simulink model "IKTrajectoryControlExamplechangepoints_MechanicalArm"  (R2019b)
settings: Solver=ode3  StartTime=0.0  StopTime=10  FixedStep=Ts  RelTol=1e-3
PostLoadFcn:
  | robot=importrobot('demo.urdf');
  | robot.DataFormat = 'column';
  | 
  | I = imread('coins.png');
  | imageOrigin = [40,20,0.08];
  | scale = .15;
model workspace (MAT data in the model file):
  I = [49 47 48 48 48 48 48 51 50 51 50 47 ... (73800 elements, 246x300)]
  Ts = 0.01
  filterConst = 0.08
  force_range = [0.8 0.9]
  imageOrigin = [0.4 0.2 0.08]
  initTargetPose = [-1  0  1.22464679915e-16  0.4; 0  1  0  0.2; -1.22464679915e-16  0  -1  0.28; 0  0  0  1]
  q0 = [0.422405030154; 0; -1.22880122285; 0]
  robot = robotics.RigidBodyTree
  robot.TreeInternal = robotics.manip.internal.RigidBodyTree
  robot.TreeInternal.NumBodies = 4
  robot.TreeInternal.Base = robotics.manip.internal.RigidBody
  robot.TreeInternal.Base.Index = 0
  robot.TreeInternal.Base.NameInternal = 'base_link'
  robot.TreeInternal.Base.JointInternal = robotics.Joint
  robot.TreeInternal.Base.JointInternal.Type = 'fixed'
  robot.TreeInternal.Base.JointInternal.VelocityNumber = 0
  robot.TreeInternal.Base.JointInternal.PositionNumber = 0
  robot.TreeInternal.Base.JointInternal.MotionSubspace = [0; 0; 0; 0; 0; 0]
  robot.TreeInternal.Base.JointInternal.NameInternal = 'base_link_jnt'
  robot.TreeInternal.Base.ParentIndex = -1
  robot.TreeInternal.Base.ChildrenIndices = 1
  robot.TreeInternal.Base.MassInternal = 60.86397744
  robot.TreeInternal.Base.CenterOfMassInternal = [0 0 0]
  robot.TreeInternal.Base.InertiaInternal = [5.0635929  0.00103417  0.80199628; 0.00103417  6.08689388  0.00105311; 0.80199628  0.00105311  4.96191932]
  robot.TreeInternal.Base.SpatialInertia = [5.0635929  0.00103417  0.80199628  0  0  0; 0.00103417  6.08689388  0.00105311  0  0  0; 0.80199628  0.00105311  4.96191932  0  0  0; 0  0  0  60.86397744  0  0; 0  0  0  0  60.86397744  0; 0  0  0  0  0  60.86397744]
  robot.TreeInternal.Base.VisualsInternal{1} = robotics.manip.internal.RigidBodyGeometry
  robot.TreeInternal.Base.VisualsInternal{1}.SourceData = {'Mesh', 'C:\Users\xxoo\Desktop\齐鹏老师\程序源码\TrajectoryControlThroughInverseKinematicsExample\magician\meshes\base_link.STL'}
  robot.TreeInternal.Base.VisualsInternal{1}.Vertices = [0.0640000030398 0.0640000030398 -0.0640000030398 -0.0640000030398 -0.0686352550983 -0.0686352550983 -0.0688218101859 -0.0640000030398 0.0686352550983 0.0640000030398 -0.0640000030398 0.0640000030398 ... (13851 elements, 4617x3)]
  robot.TreeInternal.Base.VisualsInternal{1}.Faces = [1 2 5 4 6 7 8 9 8 10 11 12 ... (28218 elements, 9406x3)]
  robot.TreeInternal.Base.VisualsInternal{1}.Color = [1 1 1 1]
  robot.TreeInternal.Base.VisualsInternal{1}.Tform = [1  0  0  0; 0  1  0  0; 0  0  1  0; 0  0  0  1]
  robot.TreeInternal.Gravity = [0 0 0]
  robot.TreeInternal.Bodies{1} = robotics.manip.internal.RigidBody
  robot.TreeInternal.Bodies{1}.Index = 1
  robot.TreeInternal.Bodies{1}.NameInternal = 'link_1'
  robot.TreeInternal.Bodies{1}.JointInternal = robotics.Joint
  robot.TreeInternal.Bodies{1}.JointInternal.Type = 'revolute'
  robot.TreeInternal.Bodies{1}.JointInternal.VelocityNumber = 1
  robot.TreeInternal.Bodies{1}.JointInternal.PositionNumber = 1
  robot.TreeInternal.Bodies{1}.JointInternal.MotionSubspace = [0; 0; 1; 0; 0; 0]
  robot.TreeInternal.Bodies{1}.JointInternal.InTree = 1
  robot.TreeInternal.Bodies{1}.JointInternal.JointToParentTransform = [1  0  0  0; 0  1  0  0; 0  0  1  0.024; 0  0  0  1]
  robot.TreeInternal.Bodies{1}.JointInternal.NameInternal = 'joint_1'
  robot.TreeInternal.Bodies{1}.JointInternal.PositionLimitsInternal = [-3.14159265 3.14159265]
  robot.TreeInternal.Bodies{1}.JointInternal.JointAxisInternal = [0 0 1]
  robot.TreeInternal.Bodies{1}.ParentIndex = 0
  robot.TreeInternal.Bodies{1}.ChildrenIndices = [0 1]
  robot.TreeInternal.Bodies{1}.MassInternal = 2.0687
  robot.TreeInternal.Bodies{1}.CenterOfMassInternal = [-0.0006241 -2.8025e-05 0.065404]
  robot.TreeInternal.Bodies{1}.InertiaInternal = [0.0156091448937  -4.20601823957e-05  8.38224731207e-05; -4.20601823957e-05  0.0156377490293  1.96798176658e-05; 8.38224731207e-05  1.96798176658e-05  0.00740390738508]
  robot.TreeInternal.Bodies{1}.SpatialInertia = [0.0156091448937  -4.20601823957e-05  8.38224731207e-05  0  -0.1353012548  -5.79753175e-05; -4.20601823957e-05  0.0156377490293  1.96798176658e-05  0.1353012548  0  0.00129107567; 8.38224731207e-05  1.96798176658e-05  0.00740390738508  5.79753175e-05  -0.00129107567  0; 0  0.1353012548  5.79753175e-05  2.0687  0  0; -0.1353012548  0  -0.00129107567  0  2.0687  0; -5.79753175e-05  0.00129107567  0  0  0  2.0687]
  robot.TreeInternal.Bodies{1}.VisualsInternal{1} = robotics.manip.internal.RigidBodyGeometry
  robot.TreeInternal.Bodies{1}.VisualsInternal{1}.SourceData = {'Mesh', 'C:\Users\xxoo\Desktop\齐鹏老师\程序源码\TrajectoryControlThroughInverseKinematicsExample\magician\meshes\link_1.STL'}
  robot.TreeInternal.Bodies{1}.VisualsInternal{1}.Vertices = [-0.0161934196949 -0.0211831368506 -0.0211831368506 -0.0161934196949 -0.0211167745292 -0.0211167745292 -0.0161065105349 0.0211831368506 -0.0083934366703 -0.0083934366703 -0.0161065105349 0.0161934196949 ... (4779 elements, 1593x3)]
  robot.TreeInternal.Bodies{1}.VisualsInternal{1}.Faces = [1 4 5 2 6 7 8 5 9 10 8 5 ... (9570 elements, 3190x3)]
  robot.TreeInternal.Bodies{1}.VisualsInternal{1}.Tform = [1  0  0  0; 0  1  0  0; 0  0  1  0; 0  0  0  1]
  robot.TreeInternal.Bodies{2} = robotics.manip.internal.RigidBody
  robot.TreeInternal.Bodies{2}.Index = 2
  robot.TreeInternal.Bodies{2}.NameInternal = 'link_2'
  robot.TreeInternal.Bodies{2}.JointInternal = robotics.Joint
  robot.TreeInternal.Bodies{2}.JointInternal.Type = 'revolute'
  robot.TreeInternal.Bodies{2}.JointInternal.VelocityNumber = 1
  robot.TreeInternal.Bodies{2}.JointInternal.PositionNumber = 1
  robot.TreeInternal.Bodies{2}.JointInternal.MotionSubspace = [0; 0; 1; 0; 0; 0]
  robot.TreeInternal.Bodies{2}.JointInternal.InTree = 1
  robot.TreeInternal.Bodies{2}.JointInternal.JointToParentTransform = [1.79489651492e-09  1.79489651492e-09  -1  -0.01175; -1  3.22165349927e-18  -1.79489651492e-09  0; 0  1  1.79489651492e-09  0.114; 0  0  0  1]
  robot.TreeInternal.Bodies{2}.JointInternal.NameInternal = 'joint_2'
  robot.TreeInternal.Bodies{2}.JointInternal.PositionLimitsInternal = [0 1.570796325]
  robot.TreeInternal.Bodies{2}.JointInternal.JointAxisInternal = [0 0 1]
  robot.TreeInternal.Bodies{2}.ParentIndex = 1
  robot.TreeInternal.Bodies{2}.ChildrenIndices = [0 0 1]
  robot.TreeInternal.Bodies{2}.MassInternal = 5.3213
  robot.TreeInternal.Bodies{2}.CenterOfMassInternal = [0.024366 0.010969 0.14363]
  robot.TreeInternal.Bodies{2}.InertiaInternal = [0.163730420845  0.00328707266887  -0.00688889284075; 0.00328707266887  0.170837433776  -0.000365688261111; -0.00688889284075  -0.000365688261111  0.0274585195056]
  robot.TreeInternal.Bodies{2}.SpatialInertia = [0.163730420845  0.00328707266887  -0.00688889284075  0  -0.764298319  0.0583693397; 0.00328707266887  0.170837433776  -0.000365688261111  0.764298319  0  -0.1296587958; -0.00688889284075  -0.000365688261111  0.0274585195056  -0.0583693397  0.1296587958  0; 0  0.764298319  -0.0583693397  5.3213  0  0; -0.764298319  0  0.1296587958  0  5.3213  0; 0.0583693397  -0.1296587958  0  0  0  5.3213]
  robot.TreeInternal.Bodies{2}.VisualsInternal{1} = robotics.manip.internal.RigidBodyGeometry
  robot.TreeInternal.Bodies{2}.VisualsInternal{1}.SourceData = {'Mesh', 'C:\Users\xxoo\Desktop\齐鹏老师\程序源码\TrajectoryControlThroughInverseKinematicsExample\magician\meshes\link_2.STL'}
  robot.TreeInternal.Bodies{2}.VisualsInternal{1}.Vertices = [0.0111309718341 0.0105486791581 0.0104152234271 0.0111560225487 0.0105787822977 0.0104152234271 0.0105787822977 0.0109527166933 0.0105486791581 0.0111309718341 0.0113159539178 0.0109527166933 ... (12384 elements, 4128x3)]
  robot.TreeInternal.Bodies{2}.VisualsInternal{1}.Faces = [1 4 5 2 6 7 1 8 9 10 9 11 ... (25242 elements, 8414x3)]
  robot.TreeInternal.Bodies{2}.VisualsInternal{1}.Tform = [1  0  0  0; 0  1  0  0; 0  0  1  0; 0  0  0  1]
  robot.TreeInternal.Bodies{3} = robotics.manip.internal.RigidBody
  robot.TreeInternal.Bodies{3}.Index = 3
  robot.TreeInternal.Bodies{3}.NameInternal = 'link_5'
  robot.TreeInternal.Bodies{3}.JointInternal = robotics.Joint
  robot.TreeInternal.Bodies{3}.JointInternal.Type = 'revolute'
  robot.TreeInternal.Bodies{3}.JointInternal.VelocityNumber = 1
  robot.TreeInternal.Bodies{3}.JointInternal.PositionNumber = 1
  robot.TreeInternal.Bodies{3}.JointInternal.MotionSubspace = [0; 0; 1; 0; 0; 0]
  robot.TreeInternal.Bodies{3}.JointInternal.InTree = 1
  robot.TreeInternal.Bodies{3}.JointInternal.JointToParentTransform = [-1  0  3.58979302984e-09  0.02699; 0  1  0  0.13228; -3.58979302984e-09  0  -1  -0.01175; 0  0  0  1]
  robot.TreeInternal.Bodies{3}.JointInternal.NameInternal = 'joint_5'
  robot.TreeInternal.Bodies{3}.JointInternal.PositionLimitsInternal = [0 1.570796325]
  robot.TreeInternal.Bodies{3}.JointInternal.JointAxisInternal = [0 0 1]
  robot.TreeInternal.Bodies{3}.ParentIndex = 2
  robot.TreeInternal.Bodies{3}.ChildrenIndices = [0 0 0 1]
  robot.TreeInternal.Bodies{3}.MassInternal = 1.0433
  robot.TreeInternal.Bodies{3}.CenterOfMassInternal = [-0.0027794 0.0076558 0.13273]
  robot.TreeInternal.Bodies{3}.InertiaInternal = [0.0313542290924  4.79298908915e-05  0.000561933554695; 4.79298908915e-05  0.0313271395102  5.50461833378e-05; 0.000561933554695  5.50461833378e-05  0.00130970870144]
  robot.TreeInternal.Bodies{3}.SpatialInertia = [0.0313542290924  4.79298908915e-05  0.000561933554695  0  -0.138477209  0.00798729614; 4.79298908915e-05  0.0313271395102  5.50461833378e-05  0.138477209  0  0.00289974802; 0.000561933554695  5.50461833378e-05  0.00130970870144  -0.00798729614  -0.00289974802  0; 0  0.138477209  -0.00798729614  1.0433  0  0; -0.138477209  0  -0.00289974802  0  1.0433  0; 0.00798729614  0.00289974802  0  0  0  1.0433]
  robot.TreeInternal.Bodies{3}.VisualsInternal{1} = robotics.manip.internal.RigidBodyGeometry
  robot.TreeInternal.Bodies{3}.VisualsInternal{1}.SourceData = {'Mesh', 'C:\Users\xxoo\Desktop\齐鹏老师\程序源码\TrajectoryControlThroughInverseKinematicsExample\magician\meshes\link_5.STL'}
  robot.TreeInternal.Bodies{3}.VisualsInternal{1}.Vertices = [0.0556930676103 0.0556930676103 0.0556161515415 0.0553730688989 0.0553730688989 0.0550332553685 0.0551596172154 0.0552206635475 0.0559755712748 0.0559755712748 0.0553503632545 0.0552016757429 ... (20082 elements, 6694x3)]
  robot.TreeInternal.Bodies{3}.VisualsInternal{1}.Faces = [1 4 2 5 6 7 8 9 1 10 11 7 ... (40728 elements, 13576x3)]
  robot.TreeInternal.Bodies{3}.VisualsInternal{1}.Tform = [1  0  0  0; 0  1  0  0; 0  0  1  0; 0  0  0  1]
  robot.TreeInternal.Bodies{4} = robotics.manip.internal.RigidBody
  robot.TreeInternal.Bodies{4}.Index = 4
  robot.TreeInternal.Bodies{4}.NameInternal = 'link_6'
  robot.TreeInternal.Bodies{4}.JointInternal = robotics.Joint
  robot.TreeInternal.Bodies{4}.JointInternal.Type = 'revolute'
  robot.TreeInternal.Bodies{4}.JointInternal.VelocityNumber = 1
  robot.TreeInternal.Bodies{4}.JointInternal.PositionNumber = 1
  robot.TreeInternal.Bodies{4}.JointInternal.MotionSubspace = [0; 0; 1; 0; 0; 0]
  robot.TreeInternal.Bodies{4}.JointInternal.InTree = 1
  robot.TreeInternal.Bodies{4}.JointInternal.JointToParentTransform = [-1  0  3.58979302984e-09  0.07431; 0  1  0  -0.12684; -3.58979302984e-09  0  -1  0; 0  0  0  1]
  robot.TreeInternal.Bodies{4}.JointInternal.NameInternal = 'joint_6'
  robot.TreeInternal.Bodies{4}.JointInternal.PositionLimitsInternal = [-3.14159265 3.14159265]
  robot.TreeInternal.Bodies{4}.JointInternal.JointAxisInternal = [0 0 1]
  robot.TreeInternal.Bodies{4}.ParentIndex = 3
  robot.TreeInternal.Bodies{4}.ChildrenIndices = [0 0 0]
  robot.TreeInternal.Bodies{4}.MassInternal = 1.5343
  robot.TreeInternal.Bodies{4}.CenterOfMassInternal = [0.0062067 -0.024291 0.075564]
  robot.TreeInternal.Bodies{4}.InertiaInternal = [0.0142732451632  0.000351341730925  -0.000666526423803; 0.000351341730925  0.0116923333652  0.00162764619775; -0.000666526423803  0.00162764619775  0.00406542385898]
  robot.TreeInternal.Bodies{4}.SpatialInertia = [0.0142732451632  0.000351341730925  -0.000666526423803  0  -0.1159378452  -0.0372696813; 0.000351341730925  0.0116923333652  0.00162764619775  0.1159378452  0  -0.00952293981; -0.000666526423803  0.00162764619775  0.00406542385898  0.0372696813  0.00952293981  0; 0  0.1159378452  0.0372696813  1.5343  0  0; -0.1159378452  0  0.00952293981  0  1.5343  0; -0.0372696813  -0.00952293981  0  0  0  1.5343]
  robot.TreeInternal.Bodies{4}.VisualsInternal{1} = robotics.manip.internal.RigidBodyGeometry
  robot.TreeInternal.Bodies{4}.VisualsInternal{1}.SourceData = {'Mesh', 'C:\Users\xxoo\Desktop\齐鹏老师\程序源码\TrajectoryControlThroughInverseKinematicsExample\magician\meshes\link_6.STL'}
  robot.TreeInternal.Bodies{4}.VisualsInternal{1}.Vertices = [-0.0349983945489 -0.0349983945489 -0.0355472825468 -0.0355472825468 -0.0360266044736 -0.0340975895524 -0.0340675376356 -0.0360266044736 -0.0364242307842 -0.0353734120727 -0.0355289839208 -0.0343938395381 ... (3897 elements, 1299x3)]
  robot.TreeInternal.Bodies{4}.VisualsInternal{1}.Faces = [1 4 5 6 7 2 8 9 6 10 11 12 ... (7818 elements, 2606x3)]
  robot.TreeInternal.Bodies{4}.VisualsInternal{1}.Color = [0.9 0.9 0.9 1]
  robot.TreeInternal.Bodies{4}.VisualsInternal{1}.Tform = [1  0  0  0; 0  1  0  0; 0  0  1  0; 0  0  0  1]
  robot.TreeInternal.NumNonFixedBodies = 4
  robot.TreeInternal.PositionNumber = 4
  robot.TreeInternal.VelocityNumber = 4
  robot.TreeInternal.PositionDoFMap = [1  1; 2  2; 3  3; 4  4]
  robot.TreeInternal.VelocityDoFMap = [1  1; 2  2; 3  3; 4  4]
  robot.TreeInternal.MaxNumBodies = 4
  robot.TreeInternal.MaxNameLength = 200
  robot.TreeInternal.MaxJointPositionNumber = 7
  robot.TreeInternal.VisualizationInfo = robotics.manip.internal.VisualizationInfo
  robot.TreeInternal.VisualizationInfo.ShowTag = 'DO_NOT_EDIT_KA8A5'
  robot.TreeInternal.DataFormatInternal = 'struct'
  scale = 0.0015
  wayPoints = [0 0 0 0 0 0 0 0 0 0 0 0 ... (1212 elements, 202x6)]
  weights = [1 1 1 1]
  weights1 = [1 1 1 1 1 1]
undefined symbols (not defined in the file or in its folder): Levenberg, Marquardt
libraries: robotmaniplib x6, simulink x2
(part 1 of 2)
settings Model: OrderedModelArguments=off  Creator=The MathWorks, Inc.  LastModifiedBy=DXQ
settings DataIOCC: SaveFormat=StructureWithTime  ReturnWorkspaceOutputs=off
settings OptimizationCC: BlockReduction=off  BufferReuse=off
settings DebuggingCC: AlgebraicLoopMsg=none  UnconnectedInputMsg=none  UnconnectedOutputMsg=none  UnconnectedLineMsg=none  PregeneratedLibrarySubsystemCodeDiagnostic=none  UnderSpecifiedDimensionMsg=warning  ArithmeticOperatorsInVariantConditions=warning
settings SFSimCC: SimUseLocalCustomCode=off  CustomCodeUndefinedFunction=UseInterfaceOnly
settings RTWCC: RTWUseLocalCustomCode=off

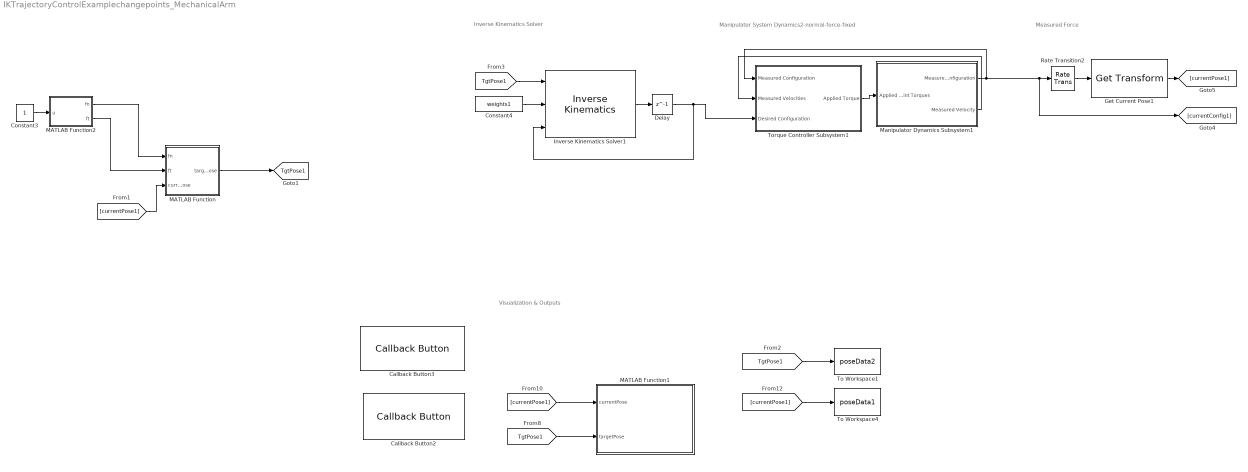
== system IKTrajectoryControlExamplechangepoints_MechanicalArm ==
  note: Visualization & Outputs
  note: Measured Force
  note: Manipulator System Dynamics2-normal-force-fixed
  note: Inverse Kinematics Solver
  Callback Button2 : CallbackButton  ButtonText=Show Image Processing Used for Waypoint Generation
      settings: ClickFcn=|
      | f1 = figure(1);
      | f1.Position = [158 253 953 335];
      | I1 = imread('coins.png');
      | I2 = imread('coinBoundaries.png');
      | 
      | subplot(1,2,1)
      | imshow(I1, 'Border', 'tight')
      | title('Original Image')
      | 
      | subplot(1,2,2)
      | imshow(I2, 'Border', 'tight')
      | title('Processed Image with Boundary Detection')
  Callback Button3 : CallbackButton  ButtonText=Visualize Model Output with Manipulator Mesh
      settings: ClickFcn=|
      | if exist('jointData1', 'var')
      |     exampleHelperVisualizeIK(I, jointData1, poseData1, sawyer, imageOrigin, scale);
      | else
      |     sim(gcs)
      |     exampleHelperVisualizeIK(I, jointData1, poseData1, sawyer, imageOrigin, scale);
      | end
  Constant3 : Constant
  Constant4 : Constant  Value=weights1
  Delay : Delay  DelayLength=1  InitialCondition=0
  Get Current Pose1 : robotmaniplib/Get Transform  RigidBodyTree=robot  SourceBody=link_6  TargetBody=base_link  SimulateUsing=Interpreted execution
      settings: SourceProductName=Robotics System Toolbox
  Inverse Kinematics Solver1 : robotmaniplib/Inverse Kinematics  RigidBodyTree=robot  EndEffector=link_6  ShowInfo=off  SolverName=Levenberg-Marquardt  EnforceJointLimits=on  MaxIterations=1500  MaxTime=10  GradientTolerance=1e-7  SolutionTolerance=1e-5  StepTolerance=1e-14  ErrorChangeTolerance=1e-8  UseErrorDamping=on  DampingBias=0.0025  SimulateUsing=Interpreted execution
      settings: SourceProductName=Robotics System Toolbox
  MATLAB Function : MATLAB Function  TreatAsAtomicUnit=on
  MATLAB Function1 : MATLAB Function  TreatAsAtomicUnit=on  SystemSampleTime=.1
  MATLAB Function2 : MATLAB Function  TreatAsAtomicUnit=on
  Manipulator Dynamics Subsystem1 : Subsystem
  Rate Transition2 : RateTransition
  To Workspace1 : ToWorkspace  VariableName=poseData2  SampleTime=-1
  To Workspace4 : ToWorkspace  VariableName=poseData1  SampleTime=-1
  Torque Controller Subsystem1 : Subsystem
  tag scope: TgtPose1=global
  wires:
  [TgtPose1] -> MATLAB Function1/2(targetPose)
  [currentPose1] -> MATLAB Function1/1(currentPose)
  [currentPose1] -> To Workspace4/1
  MATLAB Function/1(targetPose) -> [TgtPose1]
  MATLAB Function2/2(ft) -> MATLAB Function/2(ft)
  MATLAB Function2/1(fn) -> MATLAB Function/1(fn)
  Constant3/1 -> MATLAB Function2/1(u)
  [currentPose1] -> MATLAB Function/3(currentPose)
  Rate Transition2/1 -> Get Current Pose1/1
  Torque Controller Subsystem1/1(Applied Torque) -> Manipulator Dynamics Subsystem1/1(Applied Joint Torques)
  Manipulator Dynamics Subsystem1/2(Measured Velocity) -> Torque Controller Subsystem1/2(Measured Velocities)
  Constant4/1 -> Inverse Kinematics Solver1/2
  Manipulator Dynamics Subsystem1/1(Measured Configuration) -> Rate Transition2/1, [currentConfig1], Torque Controller Subsystem1/1(Measured Configuration)
  [TgtPose1] -> Inverse Kinematics Solver1/1
  [TgtPose1] -> To Workspace1/1
  Get Current Pose1/1 -> [currentPose1]
  Inverse Kinematics Solver1/1 -> Delay/1
  Delay/1 -> Torque Controller Subsystem1/3(Desired Configuration), Inverse Kinematics Solver1/3
